simulink subsystem "Visualization"  (R2021a)
settings: Solver=VariableStepAuto  StartTime=0.0  StopTime=10.0  RelTol=1e-3
model mask{animationControl=0}
  mask prompts: animationControl "Animation Control"
libraries: aerolibutil x2, vrlib x2
settings Model: Creator=luke  LastModifiedBy=csmen

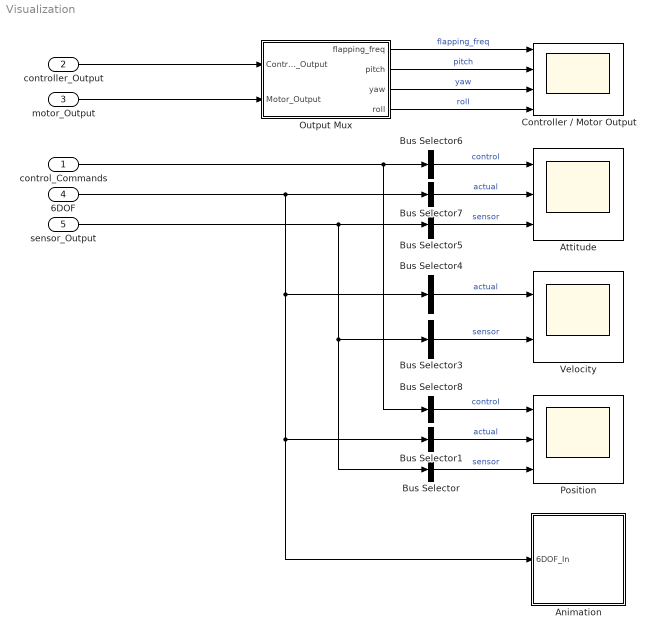
== system Visualization ==
  control_Commands : Inport
  controller_Output : Inport  Port=2
  motor_Output : Inport  Port=3
  6DOF : Inport  Port=4
  sensor_Output : Inport  Port=5
  Animation : Subsystem  Variant=on
      mask Display: disp('Animation');
  Attitude : Scope  NumInputPorts=3
  Bus Selector : BusSelector  OutputSignals=x,y,z  OutputAsBus=on
  Bus Selector1 : BusSelector  OutputSignals=inertial.position  OutputAsBus=on
  Bus Selector3 : BusSelector  OutputSignals=Vx,Vy,Vz  OutputAsBus=on
  Bus Selector4 : BusSelector  OutputSignals=inertial.velocity  OutputAsBus=on
  Bus Selector5 : BusSelector  OutputSignals=phi,theta,psi  OutputAsBus=on
  Bus Selector6 : BusSelector  OutputSignals=phi,theta,psi  OutputAsBus=on
  Bus Selector7 : BusSelector  OutputSignals=body.angles  OutputAsBus=on
  Bus Selector8 : BusSelector  OutputSignals=x,y,z  OutputAsBus=on
  Controller / Motor Output : Scope  NumInputPorts=4
  Output Mux : Subsystem
  Position : Scope  NumInputPorts=3
  Velocity : Scope  NumInputPorts=2
  wires:
  control_Commands/1 -> Bus Selector6/1, Bus Selector8/1
  Bus Selector6/1 -> Attitude/1  "control"
  Bus Selector1/1 -> Position/2  "actual"
  Output Mux/4(roll) -> Controller / Motor Output/4  "roll"
  Output Mux/2(pitch) -> Controller / Motor Output/2  "pitch"
  Bus Selector3/1 -> Velocity/2  "sensor"
  Bus Selector/1 -> Position/3  "sensor"
  Bus Selector7/1 -> Attitude/2  "actual"
  Bus Selector4/1 -> Velocity/1  "actual"
  sensor_Output/1 -> Bus Selector5/1, Bus Selector3/1, Bus Selector/1
  Output Mux/3(yaw) -> Controller / Motor Output/3  "yaw"
  Bus Selector8/1 -> Position/1  "control"
  Output Mux/1(flapping_freq) -> Controller / Motor Output/1  "flapping_freq"
  motor_Output/1 -> Output Mux/2(Motor_Output)
  controller_Output/1 -> Output Mux/1(Controller_Output)
  Bus Selector5/1 -> Attitude/3  "sensor"
  6DOF/1 -> Bus Selector7/1, Bus Selector4/1, Animation/1(6DOF_In), Bus Selector1/1

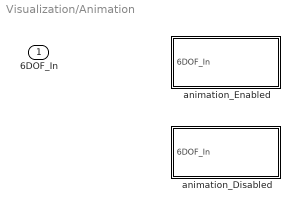
== system Visualization/Animation ==
  6DOF_In : Inport
  animation_Disabled : Subsystem  VariantControl=animationControl == 0
      mask Display: disp('Animation Disabled');
  animation_Enabled : Subsystem  VariantControl=animationControl == 1
      mask Display: disp('Animation Enabled');

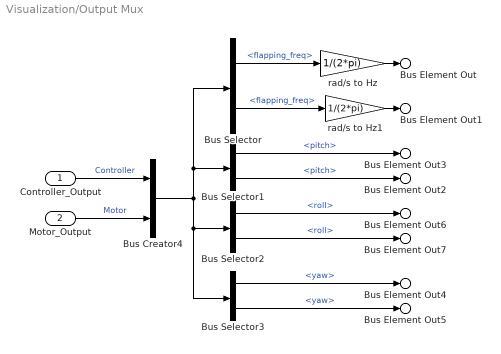
== system Visualization/Output Mux ==
  Controller_Output : Inport
  Motor_Output : Inport  Port=2
  Bus Creator4 : BusCreator  Inputs=2
  Bus Selector : BusSelector  OutputSignals=Controller.flapping_freq,Motor.flapping_freq
  Bus Selector1 : BusSelector  OutputSignals=Controller.pitch,Motor.pitch
  Bus Selector2 : BusSelector  OutputSignals=Controller.roll,Motor.roll
  Bus Selector3 : BusSelector  OutputSignals=Controller.yaw,Motor.yaw
  rad/s to Hz : Gain  Gain=1/(2*pi)
  rad/s to Hz1 : Gain  Gain=1/(2*pi)
  Bus Element Out : Outport  PortName=flapping_freq  Element=controller
  Bus Element Out1 : Outport  PortName=flapping_freq  Element=motor
  Bus Element Out2 : Outport  Port=2  PortName=pitch  Element=motor
  Bus Element Out3 : Outport  Port=2  PortName=pitch  Element=controller
  Bus Element Out4 : Outport  Port=3  PortName=yaw  Element=controller
  Bus Element Out5 : Outport  Port=3  PortName=yaw  Element=motor
  Bus Element Out6 : Outport  Port=4  PortName=roll  Element=controller
  Bus Element Out7 : Outport  Port=4  PortName=roll  Element=motor
  wires:
  rad/s to Hz1/1 -> Bus Element Out1/1
  rad/s to Hz/1 -> Bus Element Out/1
  Bus Selector3/2 -> Bus Element Out5/1  "<yaw>"
  Bus Selector3/1 -> Bus Element Out4/1  "<yaw>"
  Bus Selector2/2 -> Bus Element Out7/1  "<roll>"
  Bus Selector2/1 -> Bus Element Out6/1  "<roll>"
  Bus Selector1/2 -> Bus Element Out2/1  "<pitch>"
  Bus Selector1/1 -> Bus Element Out3/1  "<pitch>"
  Bus Selector/2 -> rad/s to Hz1/1  "<flapping_freq>"
  Bus Selector/1 -> rad/s to Hz/1  "<flapping_freq>"
  Bus Creator4/1 -> Bus Selector2/1, Bus Selector3/1, Bus Selector1/1, Bus Selector/1
  Motor_Output/1 -> Bus Creator4/2  "Motor"
  Controller_Output/1 -> Bus Creator4/1  "Controller"

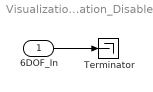
== system Visualization/Animation/animation_Disabled ==
  6DOF_In : Inport
  Terminator : Terminator
  wires:
  6DOF_In/1 -> Terminator/1

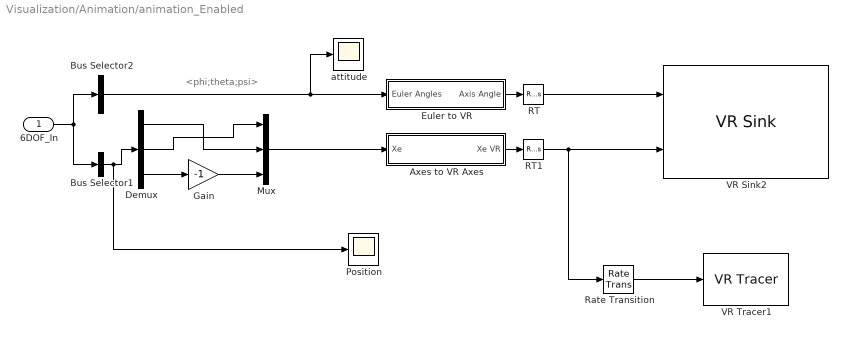
== system Visualization/Animation/animation_Enabled ==
  note: <phi;theta;psi>
  6DOF_In : Inport
  Axes to VR Axes : Subsystem
  Bus Selector1 : BusSelector  OutputSignals=inertial.position  OutputAsBus=on
  Bus Selector2 : BusSelector  OutputSignals=body.angles  OutputAsBus=on
  Demux : Demux  Outputs=3
  Euler to VR : Subsystem
  Gain : Gain  Gain=-1
  Mux : Mux  Inputs=3
  Position : Scope
  RT : RateTransition  OutPortSampleTime=0.1
  RT1 : RateTransition
  Rate Transition : RateTransition  OutPortSampleTime=1.5
  VR Sink2 : vrlib/VR Sink  InstantiateOnLoad=on  SampleTime=0.1  ViewEnable=on  RemoteChange=off  RemoteView=off  FieldsWritten=STLB_Transform.rotation.4.1.1.double#STLB_Transform.translation.3.1.1.double  WorldFileName=C:\Users\csmen\Documents\School\Fourth Year\Project\CodeRepo\MFWF-FDC\work\test2.wrl  AutoView=off  VideoDimensions=[]  AllowVariableSize=off
  VR Tracer1 : vrlib/VR Tracer  VrmlFile=C:\Users\csmen\Documents\School\Fourth Year\Project\CodeRepo\MFWF-FDC\work\test2.wrl  MarkerName=Sphere  UseLines=on  UseTriads=off  MarkerScale=[0.5 0.5 0.5]  MarkerColorSelection=Defined as RGB values  MarkerColor=red  rgbval=[1 0 0]  Ts=1.5  ForceViewerOpen=off  ConnectPlane=off  PlaneCoeff=[0 1 0 0]  ConnectPoint=None  PointCoord=[0 0 0]
      settings: SourceProductBaseCode=SL
  attitude : Scope
  wires:
  Bus Selector1/1 -> Demux/1, Position/1
  Euler to VR/1(Axis Angle) -> RT/1
  Bus Selector2/1 -> Euler to VR/1(Euler Angles), attitude/1
  Demux/1 -> Mux/2
  Axes to VR Axes/1(Xe VR) -> RT1/1
  RT1/1 -> VR Sink2/2, Rate Transition/1
  Gain/1 -> Mux/3
  Mux/1 -> Axes to VR Axes/1(Xe)
  6DOF_In/1 -> Bus Selector2/1, Bus Selector1/1
  Demux/3 -> Gain/1
  Rate Transition/1 -> VR Tracer1/1
  RT/1 -> VR Sink2/1
  Demux/2 -> Mux/1

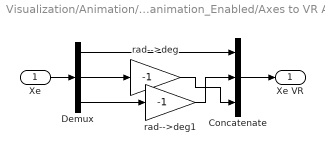
== system Visualization/Animation/animation_Enabled/Axes to VR Axes ==
  Xe : Inport
  Concatenate : Concatenate  NumInputs=3
  Demux : Demux  Outputs=3
      settings: DisplayOption=none
  rad-->deg : Gain  Gain=-1  SaturateOnIntegerOverflow=on  OutDataTypeStr=Inherit: Same as input  ParamDataTypeStr=Inherit: Same as input
  rad-->deg1 : Gain  Gain=-1  SaturateOnIntegerOverflow=on  OutDataTypeStr=Inherit: Same as input  ParamDataTypeStr=Inherit: Same as input
  Xe VR : Outport  VectorParamsAs1DForOutWhenUnconnected=off
  wires:
  rad-->deg/1 -> Concatenate/3
  rad-->deg1/1 -> Concatenate/2
  Concatenate/1 -> Xe VR/1
  Demux/3 -> rad-->deg1/1
  Demux/2 -> rad-->deg/1
  Demux/1 -> Concatenate/1
  Xe/1 -> Demux/1

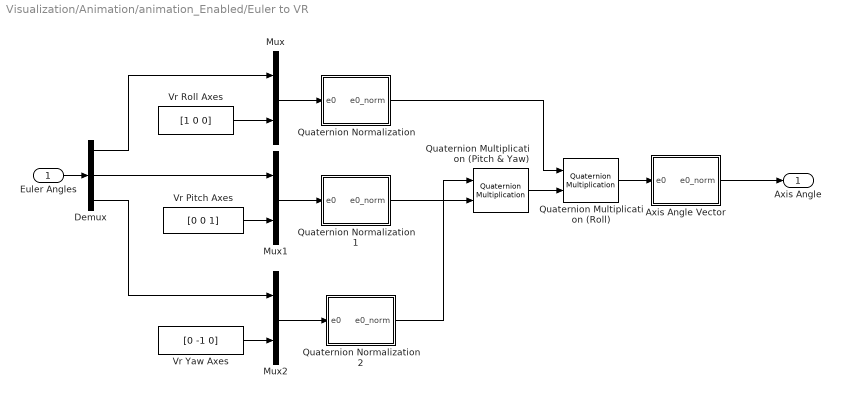
== system Visualization/Animation/animation_Enabled/Euler to VR ==
  Euler Angles : Inport
  Axis Angle Vector : Subsystem
  Demux : Demux  Outputs=3
      settings: DisplayOption=none
  Mux : Mux  Inputs=2
  Mux1 : Mux  Inputs=2
  Mux2 : Mux  Inputs=2
  Quaternion Multiplication (Pitch & Yaw) : aerolibutil/Quaternion Multiplication
  Quaternion Multiplication (Roll) : aerolibutil/Quaternion Multiplication
  Quaternion Normalization : Subsystem
  Quaternion Normalization1 : Subsystem
  Quaternion Normalization2 : Subsystem
  Vr Pitch Axes : Constant  Value=[0 0 1]
  Vr Roll Axes : Constant  Value=[1 0 0]
  Vr Yaw Axes : Constant  Value=[0 -1 0]
  Axis Angle : Outport  VectorParamsAs1DForOutWhenUnconnected=off
  wires:
  Euler Angles/1 -> Demux/1
  Vr Roll Axes/1 -> Mux/2
  Demux/1 -> Mux/1
  Vr Pitch Axes/1 -> Mux1/2
  Demux/2 -> Mux1/1
  Vr Yaw Axes/1 -> Mux2/2
  Demux/3 -> Mux2/1
  Mux/1 -> Quaternion Normalization/1(e0)
  Mux1/1 -> Quaternion Normalization1/1(e0)
  Mux2/1 -> Quaternion Normalization2/1(e0)
  Quaternion Normalization1/1(e0_norm) -> Quaternion Multiplication (Pitch & Yaw)/2
  Quaternion Normalization2/1(e0_norm) -> Quaternion Multiplication (Pitch & Yaw)/1
  Quaternion Normalization/1(e0_norm) -> Quaternion Multiplication (Roll)/1
  Axis Angle Vector/1(e0_norm) -> Axis Angle/1
  Quaternion Multiplication (Pitch & Yaw)/1 -> Quaternion Multiplication (Roll)/2
  Quaternion Multiplication (Roll)/1 -> Axis Angle Vector/1(e0)

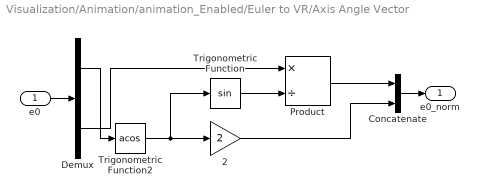
== system Visualization/Animation/animation_Enabled/Euler to VR/Axis Angle Vector ==
  e0 : Inport
  2 : Gain  Gain=2  SaturateOnIntegerOverflow=on  OutDataTypeStr=Inherit: Same as input  ParamDataTypeStr=Inherit: Same as input
  Concatenate : Concatenate
  Demux : Demux  Outputs=[1 3 ]
      settings: DisplayOption=none
  Product : Product  Inputs=*/  InputSameDT=on  SaturateOnIntegerOverflow=on  OutDataTypeStr=Inherit: Same as first input
  Trigonometric Function : Trigonometry
  Trigonometric Function2 : Trigonometry  Operator=acos
  e0_norm : Outport  VectorParamsAs1DForOutWhenUnconnected=off
  wires:
  e0/1 -> Demux/1
  Trigonometric Function2/1 -> 2/1, Trigonometric Function/1
  Trigonometric Function/1 -> Product/2
  2/1 -> Concatenate/2
  Product/1 -> Concatenate/1
  Concatenate/1 -> e0_norm/1
  Demux/2 -> Product/1
  Demux/1 -> Trigonometric Function2/1

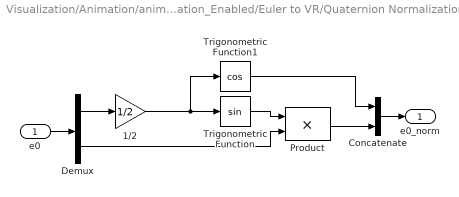
== system Visualization/Animation/animation_Enabled/Euler to VR/Quaternion Normalization ==
  e0 : Inport
  1/2 : Gain  Gain=1/2  SaturateOnIntegerOverflow=on  OutDataTypeStr=Inherit: Same as input  ParamDataTypeStr=Inherit: Same as input
  Concatenate : Concatenate
  Demux : Demux  Outputs=[1 3]
      settings: DisplayOption=none
  Product : Product  InputSameDT=on  SaturateOnIntegerOverflow=on  OutDataTypeStr=Inherit: Same as first input
  Trigonometric Function : Trigonometry
  Trigonometric Function1 : Trigonometry  Operator=cos
  e0_norm : Outport  VectorParamsAs1DForOutWhenUnconnected=off
  wires:
  e0/1 -> Demux/1
  1/2/1 -> Trigonometric Function/1, Trigonometric Function1/1
  Trigonometric Function/1 -> Product/1
  Product/1 -> Concatenate/2
  Concatenate/1 -> e0_norm/1
  Demux/1 -> 1/2/1
  Demux/2 -> Product/2
  Trigonometric Function1/1 -> Concatenate/1

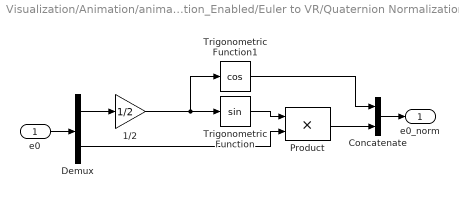
== system Visualization/Animation/animation_Enabled/Euler to VR/Quaternion Normalization1 ==
  e0 : Inport
  1/2 : Gain  Gain=1/2  SaturateOnIntegerOverflow=on  OutDataTypeStr=Inherit: Same as input  ParamDataTypeStr=Inherit: Same as input
  Concatenate : Concatenate
  Demux : Demux  Outputs=[1 3]
      settings: DisplayOption=none
  Product : Product  InputSameDT=on  SaturateOnIntegerOverflow=on  OutDataTypeStr=Inherit: Same as first input
  Trigonometric Function : Trigonometry
  Trigonometric Function1 : Trigonometry  Operator=cos
  e0_norm : Outport  VectorParamsAs1DForOutWhenUnconnected=off
  wires:
  Trigonometric Function1/1 -> Concatenate/1
  Demux/2 -> Product/2
  Demux/1 -> 1/2/1
  Concatenate/1 -> e0_norm/1
  Product/1 -> Concatenate/2
  Trigonometric Function/1 -> Product/1
  1/2/1 -> Trigonometric Function1/1, Trigonometric Function/1
  e0/1 -> Demux/1

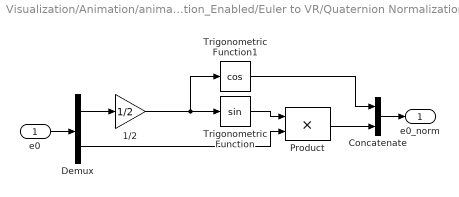
== system Visualization/Animation/animation_Enabled/Euler to VR/Quaternion Normalization2 ==
  e0 : Inport
  1/2 : Gain  Gain=1/2  SaturateOnIntegerOverflow=on  OutDataTypeStr=Inherit: Same as input  ParamDataTypeStr=Inherit: Same as input
  Concatenate : Concatenate
  Demux : Demux  Outputs=[1 3]
      settings: DisplayOption=none
  Product : Product  InputSameDT=on  SaturateOnIntegerOverflow=on  OutDataTypeStr=Inherit: Same as first input
  Trigonometric Function : Trigonometry
  Trigonometric Function1 : Trigonometry  Operator=cos
  e0_norm : Outport  VectorParamsAs1DForOutWhenUnconnected=off
  wires:
  e0/1 -> Demux/1
  1/2/1 -> Trigonometric Function/1, Trigonometric Function1/1
  Trigonometric Function/1 -> Product/1
  Product/1 -> Concatenate/2
  Concatenate/1 -> e0_norm/1
  Demux/1 -> 1/2/1
  Demux/2 -> Product/2
  Trigonometric Function1/1 -> Concatenate/1
